simulink model "simu"  (R2015a)
settings: Solver=ode45  StartTime=0.0  StopTime=10.0  FixedStep=0.01  RelTol=1e-3
values from neighbouring files (symbols this model uses):
  am = -1    [main.m]
  ap = 6/5    (= 1.2)    [main.m]
  bp = 1/5    (= 0.2)    [main.m]
  cp = -1/5    (= -0.2)    [main.m]
  ddxp0 = 0    [main.m]
  dxp0 = 0    [main.m]
  gamma = diag([100 100 100 100])    [main.m]
  km = 1    [main.m]
  kp = -1/5    (= -0.2)    [main.m]
  theta0 = [0 0 0 0]'    [main.m]
  u0 = 0    [main.m]
  xm0 = 0    [main.m]
  xp0 = 0    [main.m]
settings Model: Creator=andreas  LastModifiedBy=andreas

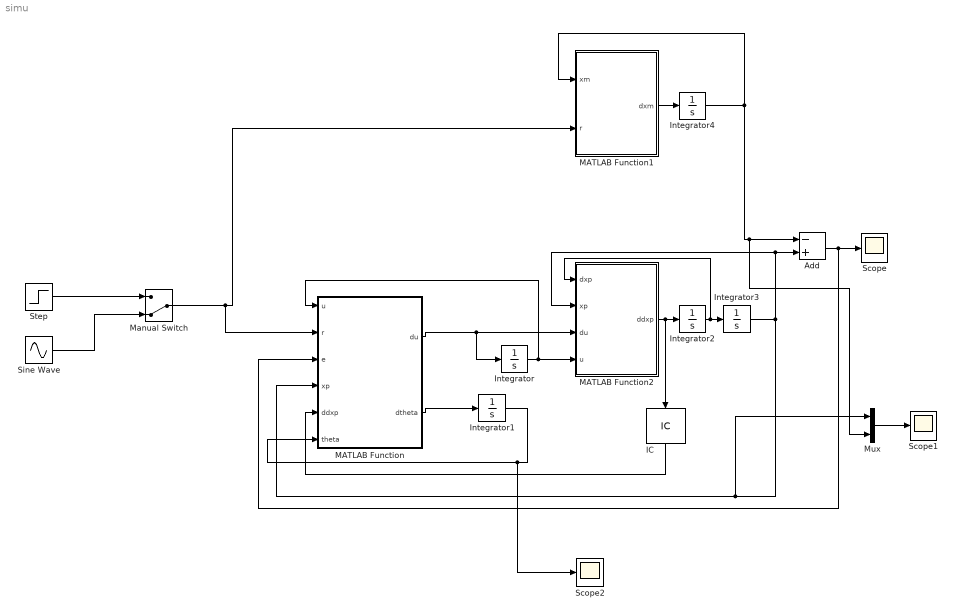
== system simu ==
  Add : Sum  Inputs=-+
  IC : InitialCondition  Value=ddxp0
  Integrator : Integrator  InitialCondition=u0
  Integrator1 : Integrator  InitialCondition=theta0
  Integrator2 : Integrator  InitialCondition=dxp0
  Integrator3 : Integrator  InitialCondition=xp0
  Integrator4 : Integrator  InitialCondition=xm0
  MATLAB Function : MATLAB Function  TreatAsAtomicUnit=on
  MATLAB Function1 : MATLAB Function  TreatAsAtomicUnit=on
  MATLAB Function2 : MATLAB Function  TreatAsAtomicUnit=on
  Manual Switch : ManualSwitch  CurrentSetting=0
  Mux : Mux  Inputs=2
  Scope : Scope
      settings: YMin=-0.35  YMax=0
  Scope1 : Scope
      settings: YMin=-0.1  YMax=0.2
  Scope2 : Scope
      settings: ShowLegends=on  YMin=-2  YMax=1.5  SaveName=ScopeData2
  Sine Wave : Sin  Amplitude=4  Frequency=2*pi/10  SampleTime=0
  Step : Step  SampleTime=0
  wires:
  MATLAB Function/1(du) -> Integrator/1, MATLAB Function2/3(du)
  Integrator/1 -> MATLAB Function/1(u), MATLAB Function2/4(u)
  MATLAB Function/2(dtheta) -> Integrator1/1
  Integrator1/1 -> Scope2/1, MATLAB Function/6(theta)
  MATLAB Function2/1(ddxp) -> IC/1, Integrator2/1
  Integrator2/1 -> MATLAB Function2/1(dxp), Integrator3/1
  Integrator3/1 -> Mux/1, MATLAB Function/4(xp), Add/2, MATLAB Function2/2(xp)
  MATLAB Function1/1(dxm) -> Integrator4/1
  Integrator4/1 -> Mux/2, Add/1, MATLAB Function1/1(xm)
  Add/1 -> Scope/1, MATLAB Function/3(e)
  IC/1 -> MATLAB Function/5(ddxp)
  Mux/1 -> Scope1/1
  Step/1 -> Manual Switch/1
  Manual Switch/1 -> MATLAB Function/2(r), MATLAB Function1/2(r)
  Sine Wave/1 -> Manual Switch/2

== matlab function simu/MATLAB Function1 ==
  data: xm input; dxm output; r input; am parameter; km parameter
function dxm = ref_model(xm, r, am, km)
%#codegen

dxm = am*xm + km*r;

== matlab function simu/MATLAB Function ==
  data: u input; du output; r input; e input; xp input; ddxp input; theta input; dtheta output; gamma parameter; kp parameter
function [du, dtheta] = controller(u, r, e, xp, ddxp, theta, gamma, kp)
%#codegen

phi = [ddxp, xp, u, r]';

%du = alpha*ddxp + beta*xp + delta*u + zeta*r;
du = theta'*phi;

dtheta = -gamma*phi*e;

== matlab function simu/MATLAB Function2 ==
  data: dxp input; xp input; du input; u input; ddxp output; bp parameter; ap parameter; cp parameter; kp parameter
function ddxp = plant(dxp, xp, du, u, bp, ap, cp, kp)
%#codegen

ddxp = (1/bp)*(dxp - ap*xp - cp*du - kp*u);
